simulink library "speedgoatlib_bce"  (R2024b)
settings: Solver=VariableStepAuto  StartTime=0.0  StopTime=10.0  RelTol=1e-3
undefined symbols (not defined in the file): BCE12, BCE_Set_init, Cell_1, Cell_10, Cell_11, Cell_12, Cell_2, Cell_3, Cell_4, Cell_5, Cell_6, Cell_7, Cell_8, Cell_9, Device_01, FIU12, sg_bce, TSE04
libraries: slrealtimeethercatlib x292, simulink x92, slrealtimeutilitieslib x24
(part 1 of 4)
settings Model: Creator=timo.straessle  LastModifiedBy=speedgoat\jenkins
settings RTWCC: GPUComputeCapability=3.5
settings ConfigComp: CovBoundaryAbsTol=1.0e-5

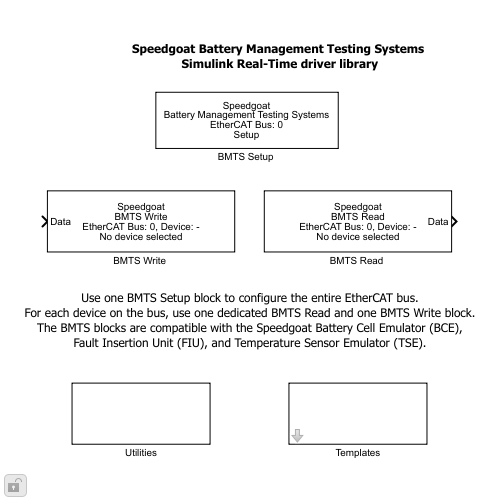
[thumbnail: Simulink's stored preview of the top-level diagram]
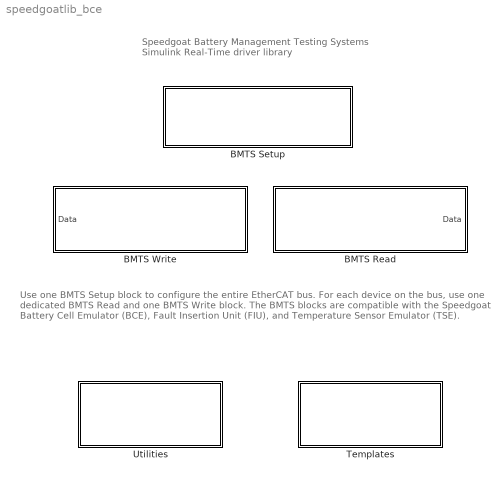
== system speedgoatlib_bce ==
  note: Speedgoat Battery Management Testing Systems
      | Simulink Real-Time driver library
  note: Use one BMTS Setup block to configure the entire EtherCAT bus.
      | For each device on the bus, use one dedicated BMTS Read and one BMTS Write block.
      | The BMTS blocks are compatible with the Speedgoat Battery Cell Emulator (BCE),
      | Fault Insertion Unit (FIU), and Temperature Sensor Emulator (TSE).
  "BMTS Read " : Subsystem  InitFcn=sg_bce.checkNumberOfBlocksGlobal(bdroot);  mask(bce_read){}
      settings: OpenFcn=sg_bce.openFcnRead;
      mask Help: eval('sg.utils.help.show(''io_main/refentry_bce_read'');')
      mask Display: disp('Speedgoat\nBMTS Read\nEtherCAT Bus: 0, Device: -\nNo device selected');port_label('output',1,'Data');
  "BMTS Setup " : Subsystem  LoadFcn=|  InitFcn=|  mask(bce_setup){}
      LoadFcn=|
      | sg_bce.createBusSignals;
      | sg_bce.setupEniCallback(gcb, bdroot);
      InitFcn=|
      | sg_bce.createBusSignals;
      | sg_bce.checkNumberOfBlocksGlobal(bdroot);
      | sg_bce.setupEniCallback(gcb, bdroot);
      settings: OpenFcn=sg_bce.openFcnSetup;
      mask Help: eval('sg.utils.help.show(''io_main/refentry_bce_setup'');')
      mask Display: disp('Speedgoat\nBattery Management Testing Systems\nEtherCAT Bus: 0\nSetup');
  "BMTS Write " : Subsystem  InitFcn=sg_bce.checkNumberOfBlocksGlobal(bdroot);  mask(bce_write){}
      settings: OpenFcn=sg_bce.openFcnWrite;
      mask Help: eval('sg.utils.help.show(''io_main/refentry_bce_write'');')
      mask Display: disp('Speedgoat\nBMTS Write\nEtherCAT Bus: 0, Device: -\nNo device selected');port_label('input',1,'Data');
  Templates : Subsystem
  Utilities : Subsystem

== system speedgoatlib_bce/BMTS Read  ==
  Subsystem : Subsystem
  Data : Outport  OutDataTypeStr=Bus: BCE_Get

== system speedgoatlib_bce/BMTS Setup  ==
  Constant : Constant
  Terminator : Terminator
  wires:
  Constant/1 -> Terminator/1

== system speedgoatlib_bce/BMTS Write  ==
  Data : Inport  OutDataTypeStr=Bus: BCE_Set
  Subsystem : Subsystem

== system speedgoatlib_bce/Templates ==
  note: These template subsystems are automatically inserted
      | by the BCE Read and Write blocks as needed.
      | Manual usage is not advised.
  "BCE AC SM Parameter Update Template " : Subsystem
  "BCE Sequencer Write Calibrate Template " : Subsystem
  "BCE Sequencer Write Template " : Subsystem
  "BCE Unit Read Calibrate Template " : Subsystem
  "BCE Unit Read Template " : Subsystem
  "BCE Unit Write Calibrate Template " : Subsystem
  "BCE Unit Write Template " : Subsystem
  "FIU Channel Read Template " : Subsystem
  "FIU Channel Write Template " : Subsystem
  "TSE Channel Read Template " : Subsystem
  "TSE Channel Write Template " : Subsystem

== system speedgoatlib_bce/Utilities ==
  "BCE AC SM Parameter Update " : Subsystem  mask(bce_ac_sm_parameter_update){}
      settings: OpenFcn=sg_bce.openFcnSeqUpdate;
      mask Help: eval('sg.utils.help.show(''io_main/refentry_bce_ac_parameter_update'');')
      mask Display: disp('Speedgoat\nBCE AC SM Parameter Update\nEtherCAT Bus: 0, Device: -\nNo device selected');port_label('input',1,'Enable');port_label('output',1,'Status');
  "BMTS Bus Pack " : Subsystem  mask(bmts_bus_pack){}
      settings: OpenFcn=sg_bce.openFcnBuspack;
      mask Help: eval('sg.utils.help.show(''io_main/refentry_bmts_buspack'');')
      mask Display: disp('Speedgoat\nBMTS\nBus Pack\nBCE12-0605');

== system speedgoatlib_bce/BMTS Read /Subsystem ==

== system speedgoatlib_bce/BMTS Write /Subsystem ==

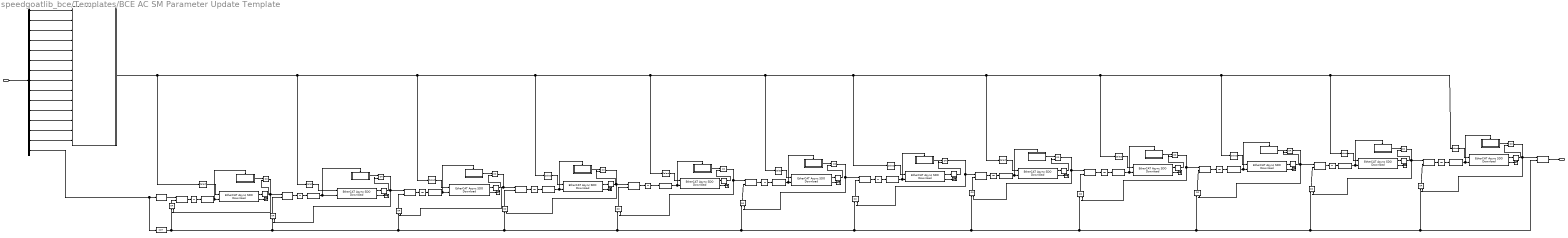
== system speedgoatlib_bce/Templates/BCE AC SM Parameter Update Template  ==
  Data : Inport
  Bus Selector : BusSelector  OutputSignals=SeqTimeStep,SeqTimeUnit,SeqOutputPath,SeqStartDelay,SeqNumCycles,SeqGainAdjustment,SeqGainSweepEnable,SeqTimeSweepEnable,SeqGainSweepUpdateTime,SeqTimeSweepUpdateTime,SeqGainSweepUpdateStep,SeqTimeSweepUpdateStep,SeqGainSweepLimitValue,SeqTimeSweepLimitValue,Enable
  Compare To Constant{,1..5,11..16} (12 alike) : simulink/Logic and Bit Operations/Compare To Constant  relop===  const=2  OutDataTypeStr=boolean
  Data Type Conversion{1..5,12..18} (12 alike) : DataTypeConversion  OutDataTypeStr=int32  SaturateOnIntegerOverflow=off  RndMeth=Floor
  Detect Increase : simulink/Logic and Bit Operations/Detect Increase  vinit=0.0  OutDataTypeStr=boolean
  Enabled Subsystem : Subsystem  TreatAsAtomicUnit=on
  Enabled Subsystem1 : Subsystem  TreatAsAtomicUnit=on
  Enabled Subsystem10 : Subsystem  TreatAsAtomicUnit=on
  Enabled Subsystem11 : Subsystem  TreatAsAtomicUnit=on
  Enabled Subsystem2 : Subsystem  TreatAsAtomicUnit=on
  Enabled Subsystem3 : Subsystem  TreatAsAtomicUnit=on
  Enabled Subsystem4 : Subsystem  TreatAsAtomicUnit=on
  Enabled Subsystem5 : Subsystem  TreatAsAtomicUnit=on
  Enabled Subsystem6 : Subsystem  TreatAsAtomicUnit=on
  Enabled Subsystem7 : Subsystem  TreatAsAtomicUnit=on
  Enabled Subsystem8 : Subsystem  TreatAsAtomicUnit=on
  Enabled Subsystem9 : Subsystem  TreatAsAtomicUnit=on
  MATLAB Function : MATLAB Function  TreatAsAtomicUnit=on
  MinMax Running Resettable{,1..12} (13 alike) : simulink/Math Operations/MinMax Running Resettable  Function=max  vinit=0.0
  NOT : Logic  Operator=NOT  AllPortsSameDT=off  OutDataTypeStr=boolean
  OR{,1..23} (24 alike) : Logic  Operator=OR  IconShape=distinctive  AllPortsSameDT=off  OutDataTypeStr=boolean
  SDO Cell 1 : slrealtimeethercatlib/EtherCAT Async SDO Download  index=0x4012  subIndex=0  sig_type=uint16  sig_dim=14  device_id=0  sample_time=0.1  subdevice_addr=0  selected_subdevice=Term 1 (EK1100)  timeout=1000  subdevice_found=1  complete=1
  SDO Cell 10 : slrealtimeethercatlib/EtherCAT Async SDO Download  index=0x401b  subIndex=0  sig_type=uint16  sig_dim=14  device_id=0  subdevice_name=Device_01 (BCE12-0605)  sample_time=0.1  subdevice_addr=1001  selected_subdevice=Term 1 (EK1100)  timeout=1000  subdevice_found=1  complete=1
  SDO Cell 11 : slrealtimeethercatlib/EtherCAT Async SDO Download  index=0x401c  subIndex=0  sig_type=uint16  sig_dim=14  device_id=0  subdevice_name=Device_01 (BCE12-0605)  sample_time=0.1  subdevice_addr=1001  selected_subdevice=Term 1 (EK1100)  timeout=1000  subdevice_found=1  complete=1
  SDO Cell 12 : slrealtimeethercatlib/EtherCAT Async SDO Download  index=0x401d  subIndex=0  sig_type=uint16  sig_dim=14  device_id=0  subdevice_name=Device_01 (BCE12-0605)  sample_time=0.1  subdevice_addr=1001  selected_subdevice=Term 1 (EK1100)  timeout=1000  subdevice_found=1  complete=1
  SDO Cell 2 : slrealtimeethercatlib/EtherCAT Async SDO Download  index=0x4013  subIndex=0  sig_type=uint16  sig_dim=14  device_id=0  subdevice_name=Device_01 (BCE12-0605)  sample_time=0.1  subdevice_addr=1001  selected_subdevice=Term 1 (EK1100)  timeout=1000  subdevice_found=1  complete=1
  SDO Cell 3 : slrealtimeethercatlib/EtherCAT Async SDO Download  index=0x4014  subIndex=0  sig_type=uint16  sig_dim=14  device_id=0  subdevice_name=Device_01 (BCE12-0605)  sample_time=0.1  subdevice_addr=1001  selected_subdevice=Term 1 (EK1100)  timeout=1000  subdevice_found=1  complete=1
  SDO Cell 4 : slrealtimeethercatlib/EtherCAT Async SDO Download  index=0x4015  subIndex=0  sig_type=uint16  sig_dim=14  device_id=0  subdevice_name=Device_01 (BCE12-0605)  sample_time=0.1  subdevice_addr=1001  selected_subdevice=Term 1 (EK1100)  timeout=1000  subdevice_found=1  complete=1
  SDO Cell 5 : slrealtimeethercatlib/EtherCAT Async SDO Download  index=0x4016  subIndex=0  sig_type=uint16  sig_dim=14  device_id=0  subdevice_name=Device_01 (BCE12-0605)  sample_time=0.1  subdevice_addr=1001  selected_subdevice=Term 1 (EK1100)  timeout=1000  subdevice_found=1  complete=1
  SDO Cell 6 : slrealtimeethercatlib/EtherCAT Async SDO Download  index=0x4017  subIndex=0  sig_type=uint16  sig_dim=14  device_id=0  subdevice_name=Device_01 (BCE12-0605)  sample_time=0.1  subdevice_addr=1001  selected_subdevice=Term 1 (EK1100)  timeout=1000  subdevice_found=1  complete=1
  SDO Cell 7 : slrealtimeethercatlib/EtherCAT Async SDO Download  index=0x4018  subIndex=0  sig_type=uint16  sig_dim=14  device_id=0  subdevice_name=Device_01 (BCE12-0605)  sample_time=0.1  subdevice_addr=1001  selected_subdevice=Term 1 (EK1100)  timeout=1000  subdevice_found=1  complete=1
  SDO Cell 8 : slrealtimeethercatlib/EtherCAT Async SDO Download  index=0x4019  subIndex=0  sig_type=uint16  sig_dim=14  device_id=0  subdevice_name=Device_01 (BCE12-0605)  sample_time=0.1  subdevice_addr=1001  selected_subdevice=Term 1 (EK1100)  timeout=1000  subdevice_found=1  complete=1
  SDO Cell 9 : slrealtimeethercatlib/EtherCAT Async SDO Download  index=0x401a  subIndex=0  sig_type=uint16  sig_dim=14  device_id=0  subdevice_name=Device_01 (BCE12-0605)  sample_time=0.1  subdevice_addr=1001  selected_subdevice=Term 1 (EK1100)  timeout=1000  subdevice_found=1  complete=1
  Selector : Selector  NumberOfDimensions=2  InputPortWidth=[12,14]  IndexOptions=Index vector (dialog),Select all  Indices=1,1  OutputSizes=1,1
  Selector1 : Selector  NumberOfDimensions=2  InputPortWidth=[12,14]  IndexOptions=Index vector (dialog),Select all  Indices=2,1  OutputSizes=1,1
  Selector10 : Selector  NumberOfDimensions=2  InputPortWidth=[12,14]  IndexOptions=Index vector (dialog),Select all  Indices=11,1  OutputSizes=1,1
  Selector11 : Selector  NumberOfDimensions=2  InputPortWidth=[12,14]  IndexOptions=Index vector (dialog),Select all  Indices=12,1  OutputSizes=1,1
  Selector2 : Selector  NumberOfDimensions=2  InputPortWidth=[12,14]  IndexOptions=Index vector (dialog),Select all  Indices=3,1  OutputSizes=1,1
  Selector3 : Selector  NumberOfDimensions=2  InputPortWidth=[12,14]  IndexOptions=Index vector (dialog),Select all  Indices=4,1  OutputSizes=1,1
  Selector4 : Selector  NumberOfDimensions=2  InputPortWidth=[12,14]  IndexOptions=Index vector (dialog),Select all  Indices=5,1  OutputSizes=1,1
  Selector5 : Selector  NumberOfDimensions=2  InputPortWidth=[12,14]  IndexOptions=Index vector (dialog),Select all  Indices=6,1  OutputSizes=1,1
  Selector6 : Selector  NumberOfDimensions=2  InputPortWidth=[12,14]  IndexOptions=Index vector (dialog),Select all  Indices=7,1  OutputSizes=1,1
  Selector7 : Selector  NumberOfDimensions=2  InputPortWidth=[12,14]  IndexOptions=Index vector (dialog),Select all  Indices=8,1  OutputSizes=1,1
  Selector8 : Selector  NumberOfDimensions=2  InputPortWidth=[12,14]  IndexOptions=Index vector (dialog),Select all  Indices=9,1  OutputSizes=1,1
  Selector9 : Selector  NumberOfDimensions=2  InputPortWidth=[12,14]  IndexOptions=Index vector (dialog),Select all  Indices=10,1  OutputSizes=1,1
  Terminator{,1..10,24} (12 alike) : Terminator
  Unit Delay{1..10,12..13} (12 alike) : UnitDelay  SampleTime=-1
  Status : Outport
  wires:
  SDO Cell 5/2 -> Terminator8/1
  OR19/1 -> OR7/2, MinMax Running Resettable8/1
  SDO Cell 7/1 -> Compare To Constant16/1
  MinMax Running Resettable10/1 -> Unit Delay9/1
  OR20/1 -> OR8/2, MinMax Running Resettable9/1
  Data Type Conversion16/1 -> Enabled Subsystem5/Enable, SDO Cell 6/2
  Selector11/1 -> SDO Cell 12/1
  Enabled Subsystem11/1(Out1) -> OR23/1
  Bus Selector/6 -> MATLAB Function/6(SeqGainAdjustment)  "<SeqGainAdjustment>"
  Bus Selector/11 -> MATLAB Function/11(SeqGainSweepUpdateStep)  "<SeqGainSweepUpdateStep>"
  MinMax Running Resettable12/1 -> Status/1
  Bus Selector/5 -> MATLAB Function/5(SeqNumCycles)  "<SeqNumCycles>"
  Selector6/1 -> SDO Cell 7/1
  Enabled Subsystem5/1(Out1) -> OR17/1
  Bus Selector/9 -> MATLAB Function/9(SeqGainSweepUpdateTime)  "<SeqGainSweepUpdateTime>"
  SDO Cell 11/2 -> Terminator3/1
  OR23/1 -> MinMax Running Resettable12/1, OR11/2
  OR3/1 -> MinMax Running Resettable3/2
  Selector4/1 -> SDO Cell 5/1
  Selector5/1 -> SDO Cell 6/1
  Compare To Constant1/1 -> OR19/2
  SDO Cell 9/2 -> Terminator/1
  Data Type Conversion14/1 -> Enabled Subsystem3/Enable, SDO Cell 4/2
  Data Type Conversion17/1 -> Enabled Subsystem6/Enable, SDO Cell 7/2
  Data Type Conversion3/1 -> Enabled Subsystem9/Enable, SDO Cell 10/2
  MinMax Running Resettable11/1 -> Unit Delay10/1
  Bus Selector/1 -> MATLAB Function/1(SeqTimeStep)  "<SeqTimeStep>"
  Enabled Subsystem7/1(Out1) -> OR19/1
  Selector7/1 -> SDO Cell 8/1
  Compare To Constant14/1 -> OR16/2
  OR9/1 -> MinMax Running Resettable9/2
  Bus Selector/2 -> MATLAB Function/2(SeqTimeUnit)  "<SeqTimeUnit>"
  MinMax Running Resettable7/1 -> Unit Delay6/1
  Bus Selector/4 -> MATLAB Function/4(SeqStartDelay)  "<SeqStartDelay>"
  OR6/1 -> MinMax Running Resettable6/2
  Compare To Constant12/1 -> OR13/2
  SDO Cell 12/1 -> Compare To Constant5/1
  OR2/1 -> MinMax Running Resettable2/2
  SDO Cell 11/1 -> Compare To Constant4/1
  Selector9/1 -> SDO Cell 10/1
  Bus Selector/14 -> MATLAB Function/14(SeqTimeSweepLimitValue)  "<SeqTimeSweepLimitValue>"
  Compare To Constant5/1 -> OR23/2
  SDO Cell 2/1 -> Compare To Constant12/1
  MinMax Running Resettable/1 -> Unit Delay13/1
  Data Type Conversion18/1 -> Enabled Subsystem7/Enable, SDO Cell 8/2
  Bus Selector/8 -> MATLAB Function/8(SeqTimeSweepEnable)  "<SeqTimeSweepEnable>"
  OR17/1 -> OR5/2, MinMax Running Resettable6/1
  OR18/1 -> OR6/2, MinMax Running Resettable7/1
  OR7/1 -> MinMax Running Resettable7/2
  MinMax Running Resettable8/1 -> Unit Delay7/1
  MinMax Running Resettable6/1 -> Unit Delay5/1
  SDO Cell 12/2 -> Terminator4/1
  Bus Selector/13 -> MATLAB Function/13(SeqGainSweepLimitValue)  "<SeqGainSweepLimitValue>"
  Compare To Constant/1 -> OR12/2
  Selector2/1 -> SDO Cell 3/1
  Data/1 -> Bus Selector/1
  Enabled Subsystem4/1(Out1) -> OR16/1
  Data Type Conversion1/1 -> Enabled Subsystem1/Enable, SDO Cell 2/2
  SDO Cell 1/1 -> Compare To Constant/1  "sdo_status"
  Data Type Conversion4/1 -> Enabled Subsystem10/Enable, SDO Cell 11/2
  Selector/1 -> SDO Cell 1/1
  MinMax Running Resettable4/1 -> Unit Delay3/1
  OR4/1 -> MinMax Running Resettable4/2
  SDO Cell 4/2 -> Terminator9/1
  OR14/1 -> MinMax Running Resettable3/1, OR2/2
  OR1/1 -> MinMax Running Resettable/2
  MATLAB Function/1(cell) -> Selector/1, Selector1/1, Selector2/1, Selector3/1, Selector4/1, Selector5/1, Selector6/1, Selector7/1, Selector8/1, Selector9/1, Selector10/1, Selector11/1
  NOT/1 -> OR/1, OR4/1, MinMax Running Resettable12/2, OR11/1, OR10/1, OR9/1, OR8/1, OR7/1, OR6/1, OR5/1, OR3/1, OR2/1, OR1/1
  OR/1 -> MinMax Running Resettable1/2
  Bus Selector/10 -> MATLAB Function/10(SeqTimeSweepUpdateTime)  "<SeqTimeSweepUpdateTime>"
  Compare To Constant15/1 -> OR17/2
  SDO Cell 6/2 -> Terminator7/1
  SDO Cell 6/1 -> Compare To Constant15/1
  Selector1/1 -> SDO Cell 2/1
  Enabled Subsystem1/1(Out1) -> OR13/1
  Compare To Constant16/1 -> OR18/2
  MinMax Running Resettable3/1 -> Unit Delay2/1
  Data Type Conversion2/1 -> Enabled Subsystem8/Enable, SDO Cell 9/2
  SDO Cell 2/2 -> Terminator1/1
  OR5/1 -> MinMax Running Resettable5/2
  SDO Cell 1/2 -> Terminator24/1  "sdo_error"
  Selector3/1 -> SDO Cell 4/1
  Selector8/1 -> SDO Cell 9/1
  SDO Cell 5/1 -> Compare To Constant14/1
  Compare To Constant4/1 -> OR22/2
  SDO Cell 10/2 -> Terminator2/1
  OR10/1 -> MinMax Running Resettable10/2
  Bus Selector/7 -> MATLAB Function/7(SeqGainSweepEnable)  "<SeqGainSweepEnable>"
  OR16/1 -> OR4/2, MinMax Running Resettable5/1
  SDO Cell 7/2 -> Terminator6/1
  SDO Cell 3/2 -> Terminator10/1
  SDO Cell 8/2 -> Terminator5/1
  Enabled Subsystem3/1(Out1) -> OR15/1
  MinMax Running Resettable9/1 -> Unit Delay8/1
  Bus Selector/12 -> MATLAB Function/12(SeqTimeSweepUpdateStep)  "<SeqTimeSweepUpdateStep>"
  OR22/1 -> OR10/2, MinMax Running Resettable11/1
  Enabled Subsystem8/1(Out1) -> OR20/1
  OR21/1 -> OR9/2, MinMax Running Resettable10/1
  MinMax Running Resettable1/1 -> Unit Delay12/1
  OR13/1 -> OR1/2, MinMax Running Resettable2/1
  Compare To Constant11/1 -> OR14/2
  Selector10/1 -> SDO Cell 11/1
  SDO Cell 8/1 -> Compare To Constant1/1
  Enabled Subsystem6/1(Out1) -> OR18/1
  OR15/1 -> OR3/2, MinMax Running Resettable4/1
  Data Type Conversion5/1 -> Enabled Subsystem11/Enable, SDO Cell 12/2
  SDO Cell 3/1 -> Compare To Constant11/1
  OR12/1 -> OR/2, MinMax Running Resettable/1
  SDO Cell 4/1 -> Compare To Constant13/1
  Compare To Constant13/1 -> OR15/2
  Enabled Subsystem/1(Out1) -> OR12/1
  MinMax Running Resettable2/1 -> Unit Delay1/1
  MinMax Running Resettable5/1 -> Unit Delay4/1
  OR11/1 -> MinMax Running Resettable11/2
  SDO Cell 10/1 -> Compare To Constant3/1
  Compare To Constant3/1 -> OR21/2
  Enabled Subsystem9/1(Out1) -> OR21/1
  Data Type Conversion15/1 -> Enabled Subsystem4/Enable, SDO Cell 5/2
  Compare To Constant2/1 -> OR20/2
  OR8/1 -> MinMax Running Resettable8/2
  Data Type Conversion12/1 -> Enabled Subsystem/Enable, SDO Cell 1/2
  Enabled Subsystem2/1(Out1) -> OR14/1
  Enabled Subsystem10/1(Out1) -> OR22/1
  Data Type Conversion13/1 -> SDO Cell 3/2, Enabled Subsystem2/Enable
  Detect Increase/1 -> MinMax Running Resettable1/1
  Bus Selector/15 -> NOT/1, Detect Increase/1  "<Enable>"
  Bus Selector/3 -> MATLAB Function/3(SeqOutputPath)  "<SeqOutputPath>"
  SDO Cell 9/1 -> Compare To Constant2/1
  Unit Delay12/1 -> Data Type Conversion12/1
  Unit Delay13/1 -> Data Type Conversion1/1
  Unit Delay1/1 -> Data Type Conversion13/1
  Unit Delay2/1 -> Data Type Conversion14/1
  Unit Delay3/1 -> Data Type Conversion15/1
  Unit Delay4/1 -> Data Type Conversion16/1
  Unit Delay5/1 -> Data Type Conversion17/1
  Unit Delay6/1 -> Data Type Conversion18/1
  Unit Delay7/1 -> Data Type Conversion2/1
  Unit Delay8/1 -> Data Type Conversion3/1
  Unit Delay9/1 -> Data Type Conversion4/1
  Unit Delay10/1 -> Data Type Conversion5/1

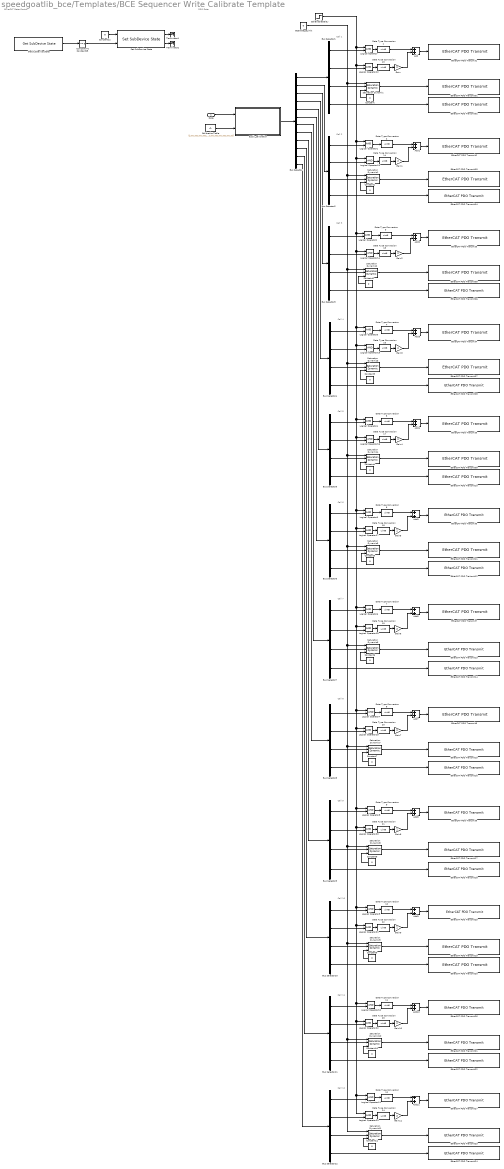
== system speedgoatlib_bce/Templates/BCE Sequencer Write Calibrate Template  ==
  note: EtherCAT State Control
  note: Cell 4
  note: Cell 8
  note: Cell 9
  note: Cell 1
  note: Cell 7
  note: PDO Data
  note: Cell 5
  note: Cell 3
  note: Cell 10
  note: Cell 6
  note: Cell 11
  note: Cell 12
  note: Cell 2
  Data : Inport  OutDataTypeStr=Bus: BCE_Set
  Add{,1..11} (12 alike) : Sum
  BceVoltageLimit : Constant  Value=6
  Bus Selector : BusSelector  OutputSignals=Cell_1,Cell_2,Cell_3,Cell_4,Cell_5,Cell_6,Cell_7,Cell_8,Cell_9,Cell_10,Cell_11,Cell_12
  Bus Selector{1..12} (12 alike) : BusSelector  OutputSignals=Enable,AC_Signal_Start,V,I
  CalibrationTable : Constant  Value=[1 0 1 0;1 0 1 0;1 0 1 0;1 0 1 0;1 0 1 0;1 0 1 0;1 0 1 0;1 0 1 0;1 0 1 0;1 0 1 0;1 0 1 0;1 0 1 0]
  CellEnableDelay : Step  Time=2  SampleTime=0
  Compare To Constant25 : simulink/Logic and Bit Operations/Compare To Constant  relop=~=  const=8  OutDataTypeStr=boolean
  Constant{,1..11} (12 alike) : Constant  Value=0
  Constant12 : Constant  Value=8  OutDataTypeStr=int32
  Data Type Conversion{1..24} (24 alike) : DataTypeConversion  OutDataTypeStr=uint8  SaturateOnIntegerOverflow=off  RndMeth=Floor
  EtherCAT PDO Transmit01 : slrealtimeethercatlib/EtherCAT PDO Transmit  Priority=3  sig_name=Device_01 (BCE12-0605).Rx_Cell_01.setVoltage  sig_offset=8  sig_type=single  type_size=32  sig_dim=1  device_id=0  sample_time=0.001000
  EtherCAT PDO Transmit02 : slrealtimeethercatlib/EtherCAT PDO Transmit  Priority=3  sig_name=Device_01 (BCE12-0605).Rx_Cell_01.setCurrent  sig_offset=40  sig_type=single  type_size=32  sig_dim=1  device_id=0  sample_time=0.001000
  EtherCAT PDO Transmit03 : slrealtimeethercatlib/EtherCAT PDO Transmit  Priority=3  sig_name=Device_01 (BCE12-0605).Rx_Cell_02.setVoltage  sig_offset=80  sig_type=single  type_size=32  sig_dim=1  device_id=0  sample_time=0.001000
  EtherCAT PDO Transmit04 : slrealtimeethercatlib/EtherCAT PDO Transmit  Priority=3  sig_name=Device_01 (BCE12-0605).Rx_Cell_02.setCurrent  sig_offset=112  sig_type=single  type_size=32  sig_dim=1  device_id=0  sample_time=0.001000
  EtherCAT PDO Transmit05 : slrealtimeethercatlib/EtherCAT PDO Transmit  Priority=3  sig_name=Device_01 (BCE12-0605).Rx_Cell_03.setVoltage  sig_offset=152  sig_type=single  type_size=32  sig_dim=1  device_id=0  sample_time=0.001000
  EtherCAT PDO Transmit06 : slrealtimeethercatlib/EtherCAT PDO Transmit  Priority=3  sig_name=Device_01 (BCE12-0605).Rx_Cell_03.setCurrent  sig_offset=184  sig_type=single  type_size=32  sig_dim=1  device_id=0  sample_time=0.001000
  EtherCAT PDO Transmit07 : slrealtimeethercatlib/EtherCAT PDO Transmit  Priority=3  sig_name=Device_01 (BCE12-0605).Rx_Cell_04.setVoltage  sig_offset=224  sig_type=single  type_size=32  sig_dim=1  device_id=0  sample_time=0.001000
  EtherCAT PDO Transmit08 : slrealtimeethercatlib/EtherCAT PDO Transmit  Priority=3  sig_name=Device_01 (BCE12-0605).Rx_Cell_04.setCurrent  sig_offset=256  sig_type=single  type_size=32  sig_dim=1  device_id=0  sample_time=0.001000
  EtherCAT PDO Transmit09 : slrealtimeethercatlib/EtherCAT PDO Transmit  Priority=3  sig_name=Device_01 (BCE12-0605).Rx_Cell_05.setVoltage  sig_offset=296  sig_type=single  type_size=32  sig_dim=1  device_id=0  sample_time=0.001000
  EtherCAT PDO Transmit1 : slrealtimeethercatlib/EtherCAT PDO Transmit  Priority=3  sig_name=Device_01 (BCE12-0605).Rx_Cell_01.enableCell  sig_offset=0  sig_type=uint8  type_size=8  sig_dim=1  device_id=0  sample_time=0.001000
  EtherCAT PDO Transmit10 : slrealtimeethercatlib/EtherCAT PDO Transmit  Priority=3  sig_name=Device_01 (BCE12-0605).Rx_Cell_05.setCurrent  sig_offset=328  sig_type=single  type_size=32  sig_dim=1  device_id=0  sample_time=0.001000
  EtherCAT PDO Transmit11 : slrealtimeethercatlib/EtherCAT PDO Transmit  Priority=3  sig_name=Device_01 (BCE12-0605).Rx_Cell_06.setVoltage  sig_offset=368  sig_type=single  type_size=32  sig_dim=1  device_id=0  sample_time=0.001000
  EtherCAT PDO Transmit12 : slrealtimeethercatlib/EtherCAT PDO Transmit  Priority=3  sig_name=Device_01 (BCE12-0605).Rx_Cell_06.setCurrent  sig_offset=400  sig_type=single  type_size=32  sig_dim=1  device_id=0  sample_time=0.001000
  EtherCAT PDO Transmit13 : slrealtimeethercatlib/EtherCAT PDO Transmit  Priority=3  sig_name=Device_01 (BCE12-0605).Rx_Cell_07.setVoltage  sig_offset=440  sig_type=single  type_size=32  sig_dim=1  device_id=0  sample_time=0.001000
  EtherCAT PDO Transmit14 : slrealtimeethercatlib/EtherCAT PDO Transmit  Priority=3  sig_name=Device_01 (BCE12-0605).Rx_Cell_07.setCurrent  sig_offset=472  sig_type=single  type_size=32  sig_dim=1  device_id=0  sample_time=0.001000
  EtherCAT PDO Transmit15 : slrealtimeethercatlib/EtherCAT PDO Transmit  Priority=3  sig_name=Device_01 (BCE12-0605).Rx_Cell_08.setVoltage  sig_offset=512  sig_type=single  type_size=32  sig_dim=1  device_id=0  sample_time=0.001000
  EtherCAT PDO Transmit16 : slrealtimeethercatlib/EtherCAT PDO Transmit  Priority=3  sig_name=Device_01 (BCE12-0605).Rx_Cell_08.setCurrent  sig_offset=544  sig_type=single  type_size=32  sig_dim=1  device_id=0  sample_time=0.001000
  EtherCAT PDO Transmit17 : slrealtimeethercatlib/EtherCAT PDO Transmit  Priority=3  sig_name=Device_01 (BCE12-0605).Rx_Cell_09.setVoltage  sig_offset=584  sig_type=single  type_size=32  sig_dim=1  device_id=0  sample_time=0.001000
  EtherCAT PDO Transmit18 : slrealtimeethercatlib/EtherCAT PDO Transmit  Priority=3  sig_name=Device_01 (BCE12-0605).Rx_Cell_09.setCurrent  sig_offset=616  sig_type=single  type_size=32  sig_dim=1  device_id=0  sample_time=0.001000
  EtherCAT PDO Transmit19 : slrealtimeethercatlib/EtherCAT PDO Transmit  Priority=3  sig_name=Device_01 (BCE12-0605).Rx_Cell_10.setVoltage  sig_offset=656  sig_type=single  type_size=32  sig_dim=1  device_id=0  sample_time=0.001000
  EtherCAT PDO Transmit2 : slrealtimeethercatlib/EtherCAT PDO Transmit  Priority=3  sig_name=Device_01 (BCE12-0605).Rx_Cell_02.enableCell  sig_offset=72  sig_type=uint8  type_size=8  sig_dim=1  device_id=0  sample_time=0.001000
  EtherCAT PDO Transmit20 : slrealtimeethercatlib/EtherCAT PDO Transmit  Priority=3  sig_name=Device_01 (BCE12-0605).Rx_Cell_10.setCurrent  sig_offset=688  sig_type=single  type_size=32  sig_dim=1  device_id=0  sample_time=0.001000
  EtherCAT PDO Transmit21 : slrealtimeethercatlib/EtherCAT PDO Transmit  Priority=3  sig_name=Device_01 (BCE12-0605).Rx_Cell_11.setVoltage  sig_offset=728  sig_type=single  type_size=32  sig_dim=1  device_id=0  sample_time=0.001000
  EtherCAT PDO Transmit22 : slrealtimeethercatlib/EtherCAT PDO Transmit  Priority=3  sig_name=Device_01 (BCE12-0605).Rx_Cell_11.setCurrent  sig_offset=760  sig_type=single  type_size=32  sig_dim=1  device_id=0  sample_time=0.001000
  EtherCAT PDO Transmit23 : slrealtimeethercatlib/EtherCAT PDO Transmit  Priority=3  sig_name=Device_01 (BCE12-0605).Rx_Cell_12.setVoltage  sig_offset=800  sig_type=single  type_size=32  sig_dim=1  device_id=0  sample_time=0.001000
  EtherCAT PDO Transmit24 : slrealtimeethercatlib/EtherCAT PDO Transmit  Priority=3  sig_name=Device_01 (BCE12-0605).Rx_Cell_12.setCurrent  sig_offset=832  sig_type=single  type_size=32  sig_dim=1  device_id=0  sample_time=0.001000
  EtherCAT PDO Transmit25 : slrealtimeethercatlib/EtherCAT PDO Transmit  Priority=3  sig_name=Device_01 (BCE12-0605).Rx_Cell_10.enableCell  sig_offset=648  sig_type=uint8  type_size=8  sig_dim=1  device_id=0  sample_time=0.001000
  EtherCAT PDO Transmit26 : slrealtimeethercatlib/EtherCAT PDO Transmit  Priority=3  sig_name=Device_01 (BCE12-0605).Rx_Cell_11.enableCell  sig_offset=720  sig_type=uint8  type_size=8  sig_dim=1  device_id=0  sample_time=0.001000
  EtherCAT PDO Transmit27 : slrealtimeethercatlib/EtherCAT PDO Transmit  Priority=3  sig_name=Device_01 (BCE12-0605).Rx_Cell_12.enableCell  sig_offset=792  sig_type=uint8  type_size=8  sig_dim=1  device_id=0  sample_time=0.001000
  EtherCAT PDO Transmit3 : slrealtimeethercatlib/EtherCAT PDO Transmit  Priority=3  sig_name=Device_01 (BCE12-0605).Rx_Cell_03.enableCell  sig_offset=144  sig_type=uint8  type_size=8  sig_dim=1  device_id=0  sample_time=0.001000
  EtherCAT PDO Transmit4 : slrealtimeethercatlib/EtherCAT PDO Transmit  Priority=3  sig_name=Device_01 (BCE12-0605).Rx_Cell_04.enableCell  sig_offset=216  sig_type=uint8  type_size=8  sig_dim=1  device_id=0  sample_time=0.001000
  EtherCAT PDO Transmit5 : slrealtimeethercatlib/EtherCAT PDO Transmit  Priority=3  sig_name=Device_01 (BCE12-0605).Rx_Cell_05.enableCell  sig_offset=288  sig_type=uint8  type_size=8  sig_dim=1  device_id=0  sample_time=0.001000
  EtherCAT PDO Transmit6 : slrealtimeethercatlib/EtherCAT PDO Transmit  Priority=3  sig_name=Device_01 (BCE12-0605).Rx_Cell_06.enableCell  sig_offset=360  sig_type=uint8  type_size=8  sig_dim=1  device_id=0  sample_time=0.001000
  EtherCAT PDO Transmit7 : slrealtimeethercatlib/EtherCAT PDO Transmit  Priority=3  sig_name=Device_01 (BCE12-0605).Rx_Cell_07.enableCell  sig_offset=432  sig_type=uint8  type_size=8  sig_dim=1  device_id=0  sample_time=0.001000
  EtherCAT PDO Transmit8 : slrealtimeethercatlib/EtherCAT PDO Transmit  Priority=3  sig_name=Device_01 (BCE12-0605).Rx_Cell_08.enableCell  sig_offset=504  sig_type=uint8  type_size=8  sig_dim=1  device_id=0  sample_time=0.001000
  EtherCAT PDO Transmit9 : slrealtimeethercatlib/EtherCAT PDO Transmit  Priority=3  sig_name=Device_01 (BCE12-0605).Rx_Cell_09.enableCell  sig_offset=576  sig_type=uint8  type_size=8  sig_dim=1  device_id=0  sample_time=0.001000
  Gain{,1..11} (12 alike) : Gain  Gain=2  OutDataTypeStr=uint8
  Get SubDevice State : slrealtimeethercatlib/Get SubDevice State  device_id=0  sample_time=1  subdevice_addr=0  selected_subdevice=Term 1 (EK1100)  timeout=500  subdevice_found=0
  Logical Operator{,1..23} (24 alike) : Logic  AllPortsSameDT=off  OutDataTypeStr=boolean
  Saturation Dynamic{,1..11} (12 alike) : simulink/Discontinuities/Saturation Dynamic  OutMin=[]  OutMax=[]  OutDataTypeStr=Inherit: Same as second input  OutDataType=fixdt(1, 16)  OutScaling=2^-10  DoSatur=off
  Set SubDevice State : slrealtimeethercatlib/Set SubDevice State  device_id=0  sample_time=1  subdevice_addr=0  selected_subdevice=Term 1 (EK1100)  subdevice_found=0
  Terminator1 : Terminator
  Terminator2 : Terminator
  apply_calibration : Subsystem
  wires:
  apply_calibration/1(bceBusOut) -> Bus Selector/1
  Data/1 -> apply_calibration/1(bceBusIn)
  CalibrationTable/1 -> apply_calibration/2(correctionTable)
  Logical Operator11/1 -> Data Type Conversion12/1
  Bus Selector12/1 -> Logical Operator11/2  "<Enable>"
  Logical Operator10/1 -> Data Type Conversion11/1
  Bus Selector11/1 -> Logical Operator10/2  "<Enable>"
  Logical Operator9/1 -> Data Type Conversion10/1
  Bus Selector10/1 -> Logical Operator9/2  "<Enable>"
  Logical Operator8/1 -> Data Type Conversion9/1
  Bus Selector9/1 -> Logical Operator8/2  "<Enable>"
  Logical Operator7/1 -> Data Type Conversion8/1
  Bus Selector8/1 -> Logical Operator7/2  "<Enable>"
  Logical Operator6/1 -> Data Type Conversion7/1
  Bus Selector7/1 -> Logical Operator6/2  "<Enable>"
  Logical Operator5/1 -> Data Type Conversion6/1
  Bus Selector6/1 -> Logical Operator5/2  "<Enable>"
  Logical Operator4/1 -> Data Type Conversion5/1
  Bus Selector5/1 -> Logical Operator4/2  "<Enable>"
  Logical Operator3/1 -> Data Type Conversion4/1
  Bus Selector4/1 -> Logical Operator3/2  "<Enable>"
  Logical Operator2/1 -> Data Type Conversion3/1
  Bus Selector3/1 -> Logical Operator2/2  "<Enable>"
  Logical Operator1/1 -> Data Type Conversion2/1
  Bus Selector2/1 -> Logical Operator1/2  "<Enable>"
  Logical Operator/1 -> Data Type Conversion1/1
  Bus Selector1/1 -> Logical Operator/2  "<Enable>"
  Constant12/1 -> Set SubDevice State/1
  Compare To Constant25/1 -> Set SubDevice State/2
  Set SubDevice State/1 -> Terminator1/1
  Set SubDevice State/2 -> Terminator2/1
  Get SubDevice State/1 -> Compare To Constant25/1
  Saturation Dynamic11/1 -> EtherCAT PDO Transmit23/1
  Constant11/1 -> Saturation Dynamic11/3
  Saturation Dynamic10/1 -> EtherCAT PDO Transmit21/1
  Constant10/1 -> Saturation Dynamic10/3
  Saturation Dynamic9/1 -> EtherCAT PDO Transmit19/1
  Constant9/1 -> Saturation Dynamic9/3
  Saturation Dynamic8/1 -> EtherCAT PDO Transmit17/1
  Constant8/1 -> Saturation Dynamic8/3
  Saturation Dynamic7/1 -> EtherCAT PDO Transmit15/1
  Constant7/1 -> Saturation Dynamic7/3
  Saturation Dynamic6/1 -> EtherCAT PDO Transmit13/1
  Constant6/1 -> Saturation Dynamic6/3
  Saturation Dynamic5/1 -> EtherCAT PDO Transmit11/1
  Constant5/1 -> Saturation Dynamic5/3
  Saturation Dynamic4/1 -> EtherCAT PDO Transmit09/1
  Constant4/1 -> Saturation Dynamic4/3
  Saturation Dynamic3/1 -> EtherCAT PDO Transmit07/1
  Constant3/1 -> Saturation Dynamic3/3
  Saturation Dynamic2/1 -> EtherCAT PDO Transmit05/1
  Constant2/1 -> Saturation Dynamic2/3
  Saturation Dynamic1/1 -> EtherCAT PDO Transmit03/1
  Constant1/1 -> Saturation Dynamic1/3
  BceVoltageLimit/1 -> Saturation Dynamic1/1, Saturation Dynamic5/1, Saturation Dynamic11/1, Saturation Dynamic10/1, Saturation Dynamic9/1, Saturation Dynamic8/1, Saturation Dynamic7/1, Saturation Dynamic6/1, Saturation Dynamic4/1, Saturation Dynamic3/1, Saturation Dynamic2/1, Saturation Dynamic/1
  Constant/1 -> Saturation Dynamic/3
  Saturation Dynamic/1 -> EtherCAT PDO Transmit01/1
  Bus Selector6/4 -> EtherCAT PDO Transmit12/1  "<I>"
  Bus Selector/4 -> Bus Selector4/1  "<Cell_4>"
  Data Type Conversion7/1 -> Add6/1
  Bus Selector11/4 -> EtherCAT PDO Transmit22/1  "<I>"
  Bus Selector9/4 -> EtherCAT PDO Transmit18/1  "<I>"
  Bus Selector/8 -> Bus Selector8/1  "<Cell_8>"
  Bus Selector8/3 -> Saturation Dynamic7/2  "<V>"
  Bus Selector5/3 -> Saturation Dynamic4/2  "<V>"
  Data Type Conversion11/1 -> Add10/1
  Bus Selector5/4 -> EtherCAT PDO Transmit10/1  "<I>"
  Bus Selector10/4 -> EtherCAT PDO Transmit20/1  "<I>"
  Bus Selector/11 -> Bus Selector11/1  "<Cell_11>"
  Bus Selector3/3 -> Saturation Dynamic2/2  "<V>"
  Bus Selector2/4 -> EtherCAT PDO Transmit04/1  "<I>"
  Bus Selector10/3 -> Saturation Dynamic9/2  "<V>"
  Bus Selector12/4 -> EtherCAT PDO Transmit24/1  "<I>"
  Bus Selector/5 -> Bus Selector5/1  "<Cell_5>"
  Bus Selector/10 -> Bus Selector10/1  "<Cell_10>"
  Bus Selector1/4 -> EtherCAT PDO Transmit02/1  "<I>"
  Data Type Conversion3/1 -> Add2/1
  Bus Selector4/3 -> Saturation Dynamic3/2  "<V>"
  Bus Selector6/3 -> Saturation Dynamic5/2  "<V>"
  Bus Selector3/4 -> EtherCAT PDO Transmit06/1  "<I>"
  Bus Selector/12 -> Bus Selector12/1  "<Cell_12>"
  Bus Selector4/4 -> EtherCAT PDO Transmit08/1  "<I>"
  Data Type Conversion1/1 -> Add/1
  Data Type Conversion10/1 -> Add9/1
  Data Type Conversion12/1 -> Add11/1
  Data Type Conversion5/1 -> Add4/1
  Data Type Conversion9/1 -> Add8/1
  Data Type Conversion6/1 -> Add5/1
  Data Type Conversion4/1 -> Add3/1
  Bus Selector/9 -> Bus Selector9/1  "<Cell_9>"
  Bus Selector7/4 -> EtherCAT PDO Transmit14/1  "<I>"
  Bus Selector7/3 -> Saturation Dynamic6/2  "<V>"
  Data Type Conversion2/1 -> Add1/1
  Bus Selector/6 -> Bus Selector6/1  "<Cell_6>"
  Bus Selector/2 -> Bus Selector2/1  "<Cell_2>"
  Bus Selector1/3 -> Saturation Dynamic/2  "<V>"
  Bus Selector/3 -> Bus Selector3/1  "<Cell_3>"
  Bus Selector8/4 -> EtherCAT PDO Transmit16/1  "<I>"
  Bus Selector/1 -> Bus Selector1/1  "<Cell_1>"
  Bus Selector11/3 -> Saturation Dynamic10/2  "<V>"
  Bus Selector/7 -> Bus Selector7/1  "<Cell_7>"
  Bus Selector2/3 -> Saturation Dynamic1/2  "<V>"
  Bus Selector12/3 -> Saturation Dynamic11/2  "<V>"
  Bus Selector9/3 -> Saturation Dynamic8/2  "<V>"
  Data Type Conversion8/1 -> Add7/1
  Bus Selector1/2 -> Logical Operator12/2  "<AC_Signal_Start>"
  Logical Operator12/1 -> Data Type Conversion13/1
  Data Type Conversion13/1 -> Gain/1
  Add/1 -> EtherCAT PDO Transmit1/1
  Gain/1 -> Add/2
  Gain1/1 -> Add1/2
  Logical Operator13/1 -> Data Type Conversion14/1
  Data Type Conversion14/1 -> Gain1/1
  Bus Selector2/2 -> Logical Operator13/2  "<AC_Signal_Start>"
  Add1/1 -> EtherCAT PDO Transmit2/1
  Gain2/1 -> Add2/2
  Data Type Conversion15/1 -> Gain2/1
  Bus Selector3/2 -> Logical Operator14/2  "<AC_Signal_Start>"
  Logical Operator14/1 -> Data Type Conversion15/1
  Add2/1 -> EtherCAT PDO Transmit3/1
  Logical Operator15/1 -> Data Type Conversion16/1
  Data Type Conversion16/1 -> Gain3/1
  Gain3/1 -> Add3/2
  Bus Selector4/2 -> Logical Operator15/2  "<AC_Signal_Start>"
  Add3/1 -> EtherCAT PDO Transmit4/1
  Bus Selector5/2 -> Logical Operator16/2  "<AC_Signal_Start>"
  Gain4/1 -> Add4/2
  Data Type Conversion17/1 -> Gain4/1
  Logical Operator16/1 -> Data Type Conversion17/1
  Add4/1 -> EtherCAT PDO Transmit5/1
  Logical Operator17/1 -> Data Type Conversion18/1
  Data Type Conversion18/1 -> Gain5/1
  Gain5/1 -> Add5/2
  Bus Selector6/2 -> Logical Operator17/2  "<AC_Signal_Start>"
  Add5/1 -> EtherCAT PDO Transmit6/1
  Logical Operator18/1 -> Data Type Conversion19/1
  Data Type Conversion19/1 -> Gain6/1
  Gain6/1 -> Add6/2
  Bus Selector7/2 -> Logical Operator18/2  "<AC_Signal_Start>"
  Add6/1 -> EtherCAT PDO Transmit7/1
  Logical Operator19/1 -> Data Type Conversion20/1
  Data Type Conversion20/1 -> Gain7/1
  Gain7/1 -> Add7/2
  Bus Selector8/2 -> Logical Operator19/2  "<AC_Signal_Start>"
  Add7/1 -> EtherCAT PDO Transmit8/1
  Logical Operator20/1 -> Data Type Conversion21/1
  Data Type Conversion21/1 -> Gain8/1
  Gain8/1 -> Add8/2
  Bus Selector9/2 -> Logical Operator20/2  "<AC_Signal_Start>"
  Add8/1 -> EtherCAT PDO Transmit9/1
  Logical Operator21/1 -> Data Type Conversion22/1
  Data Type Conversion22/1 -> Gain9/1
  Gain9/1 -> Add9/2
  Bus Selector10/2 -> Logical Operator21/2  "<AC_Signal_Start>"
  Add9/1 -> EtherCAT PDO Transmit25/1
  Logical Operator22/1 -> Data Type Conversion23/1
  Data Type Conversion23/1 -> Gain10/1
  Gain10/1 -> Add10/2
  Bus Selector11/2 -> Logical Operator22/2  "<AC_Signal_Start>"
  Add10/1 -> EtherCAT PDO Transmit26/1
  CellEnableDelay/1 -> Logical Operator/1, Logical Operator12/1, Logical Operator14/1, Logical Operator15/1, Logical Operator16/1, Logical Operator5/1, Logical Operator17/1, Logical Operator18/1, Logical Operator19/1, Logical Operator8/1, Logical Operator20/1, Logical Operator10/1, Logical Operator22/1, Logical Operator23/1, Logical Operator11/1, Logical Operator21/1, Logical Operator9/1, Logical Operator7/1, Logical Operator6/1, Logical Operator4/1, Logical Operator3/1, Logical Operator2/1, Logical Operator13/1, Logical Operator1/1
  Logical Operator23/1 -> Data Type Conversion24/1
  Data Type Conversion24/1 -> Gain11/1
  Gain11/1 -> Add11/2
  Bus Selector12/2 -> Logical Operator23/2  "<AC_Signal_Start>"
  Add11/1 -> EtherCAT PDO Transmit27/1
